simulink model "bf_ranger_indi"  (R2021a)
settings: Solver=VariableStepAuto  StartTime=0.0  StopTime=5  RelTol=1e-3
values from neighbouring files (symbols this model uses):
  am = 0.025    [ranger_sim.m]
  as = 0.08    [ranger_sim.m]
  G = [-10.67  10.67  0     0     0     0 0 ... (first row only)    [ranger_sim.m]
  G_inv = pinv(G)    [ranger_sim.m]
  G_thrust = [0 0 0 0 0 0 0 ... (first row only)    [ranger_sim.m]
  H_discr_den = cell2mat(Hd.den)    [ranger_sim.m]
  H_discr_num = cell2mat(Hd.num)    [ranger_sim.m]
  Kd = [10; 18; 18]    [ranger_sim.m]
  Kp = [4.1089; 4.7304; 7.36]    [ranger_sim.m]
  sample_time = 1/500    (= 0.002)    [ranger_sim.m]
undefined symbols (not defined in the file or in its folder): DiscIntNeverNeededParam
settings Model: Creator=AutomZ2-RG02B04  LastModifiedBy=AutomZ2-RG02A02
settings SolverCC: AlgebraicLoopSolver=TrustRegion

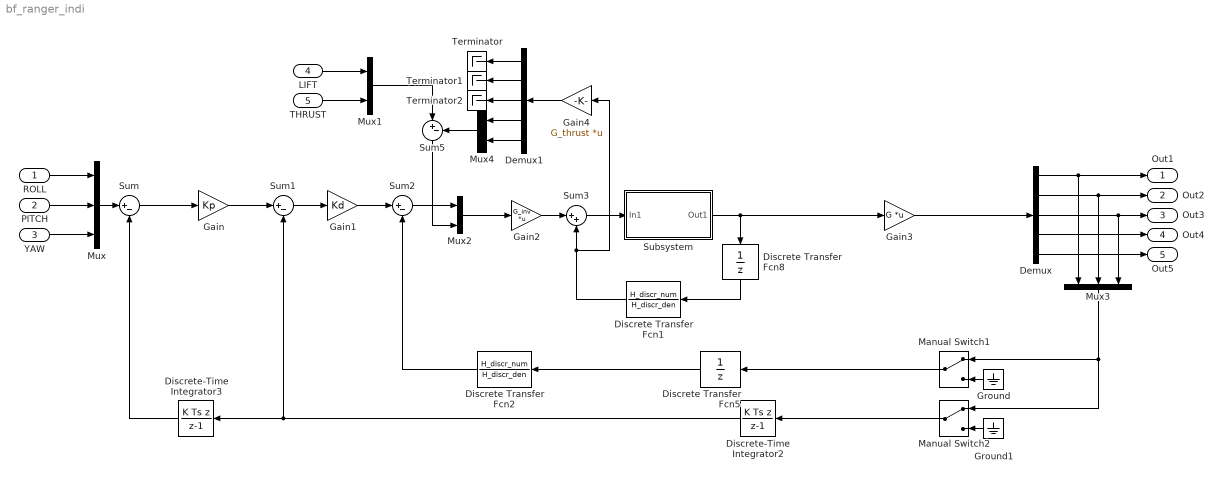
== system bf_ranger_indi ==
  ROLL : Inport
  PITCH : Inport  Port=2
  YAW : Inport  Port=3
  LIFT : Inport  Port=4
  THRUST : Inport  Port=5
  Demux : Demux  Outputs=5
  Demux1 : Demux  Outputs=5
  Discrete Transfer Fcn1 : DiscreteTransferFcn  Numerator=H_discr_num  Denominator=H_discr_den  SampleTime=sample_time
  Discrete Transfer Fcn2 : DiscreteTransferFcn  Numerator=H_discr_num  Denominator=H_discr_den  SampleTime=sample_time
  Discrete Transfer Fcn5 : DiscreteTransferFcn  Denominator=[1 0]  SampleTime=sample_time
  Discrete Transfer Fcn8 : DiscreteTransferFcn  Denominator=[1 0]  SampleTime=sample_time
  Discrete-Time Integrator2 : DiscreteIntegrator  IntegratorMethod=Integration: Backward Euler  SampleTime=sample_time  ICPrevOutput=DiscIntNeverNeededParam  ICPrevScaledInput=DiscIntNeverNeededParam
  Discrete-Time Integrator3 : DiscreteIntegrator  IntegratorMethod=Integration: Backward Euler  SampleTime=sample_time  ICPrevOutput=DiscIntNeverNeededParam  ICPrevScaledInput=DiscIntNeverNeededParam
  Gain : Gain  Gain=Kp
  Gain1 : Gain  Gain=Kd
  Gain2 : Gain  Gain=G_inv  Multiplication=Matrix(K*u)
  Gain3 : Gain  Gain=G  Multiplication=Matrix(K*u)
  Gain4 : Gain  Gain=G_thrust  Multiplication=Matrix(K*u)
  Ground : Ground
  Ground1 : Ground
  Manual Switch1 : ManualSwitch
  Manual Switch2 : ManualSwitch
  Mux : Mux  Inputs=3
  Mux1 : Mux  Inputs=2
  Mux2 : Mux  Inputs=2
  Mux3 : Mux  Inputs=3
  Mux4 : Mux  Inputs=2
  Subsystem : Subsystem
  Sum{,1..2,5} (4 alike) : Sum  Inputs=|+-
  Sum3 : Sum  Inputs=|++
  Terminator : Terminator
  Terminator1 : Terminator
  Terminator2 : Terminator
  Out1 : Outport
  Out2 : Outport  Port=2
  Out3 : Outport  Port=3
  Out4 : Outport  Port=4
  Out5 : Outport  Port=5
  wires:
  Sum/1 -> Gain/1
  Gain/1 -> Sum1/1
  Sum1/1 -> Gain1/1
  Gain1/1 -> Sum2/1
  Sum2/1 -> Mux2/1
  Gain2/1 -> Sum3/1
  Discrete Transfer Fcn5/1 -> Discrete Transfer Fcn2/1
  Discrete Transfer Fcn8/1 -> Discrete Transfer Fcn1/1
  Mux2/1 -> Gain2/1
  Sum3/1 -> Subsystem/1(In1)
  PITCH/1 -> Mux/2
  YAW/1 -> Mux/3
  Mux/1 -> Sum/1
  LIFT/1 -> Mux1/1
  THRUST/1 -> Mux1/2
  Demux/1 -> Mux3/1, Out1/1
  Demux/2 -> Mux3/2, Out2/1
  Demux/3 -> Out3/1, Mux3/3
  Demux/4 -> Out4/1
  Demux/5 -> Out5/1
  ROLL/1 -> Mux/1
  Subsystem/1(Out1) -> Discrete Transfer Fcn8/1, Gain3/1
  Gain3/1 -> Demux/1
  Discrete Transfer Fcn2/1 -> Sum2/2
  Discrete-Time Integrator2/1 -> Discrete-Time Integrator3/1, Sum1/2
  Discrete-Time Integrator3/1 -> Sum/2
  Discrete Transfer Fcn1/1 -> Gain4/1, Sum3/2
  Mux1/1 -> Sum5/1
  Sum5/1 -> Mux2/2
  Manual Switch1/1 -> Discrete Transfer Fcn5/1
  Manual Switch2/1 -> Discrete-Time Integrator2/1
  Mux3/1 -> Manual Switch2/1, Manual Switch1/1
  Ground/1 -> Manual Switch1/2
  Ground1/1 -> Manual Switch2/2
  Demux1/3 -> Terminator2/1
  Demux1/4 -> Mux4/1
  Demux1/2 -> Terminator1/1
  Gain4/1 -> Demux1/1
  Mux4/1 -> Sum5/2
  Demux1/5 -> Mux4/2
  Demux1/1 -> Terminator/1

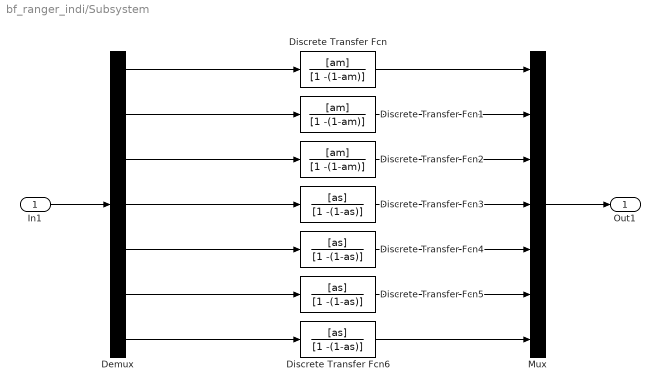
== system bf_ranger_indi/Subsystem ==
  In1 : Inport
  Demux : Demux  Outputs=7
  Discrete Transfer Fcn : DiscreteTransferFcn  Numerator=[am]  Denominator=[1 -(1-am)]  SampleTime=sample_time
  Discrete Transfer Fcn1 : DiscreteTransferFcn  Numerator=[am]  Denominator=[1 -(1-am)]
  Discrete Transfer Fcn2 : DiscreteTransferFcn  Numerator=[am]  Denominator=[1 -(1-am)]
  Discrete Transfer Fcn{3..6} (4 alike) : DiscreteTransferFcn  Numerator=[as]  Denominator=[1 -(1-as)]
  Mux : Mux  Inputs=7
  Out1 : Outport
  wires:
  Discrete Transfer Fcn/1 -> Mux/1
  Discrete Transfer Fcn1/1 -> Mux/2
  Demux/2 -> Discrete Transfer Fcn1/1
  Discrete Transfer Fcn2/1 -> Mux/3
  Demux/3 -> Discrete Transfer Fcn2/1
  Demux/5 -> Discrete Transfer Fcn4/1
  Discrete Transfer Fcn3/1 -> Mux/4
  Demux/4 -> Discrete Transfer Fcn3/1
  Discrete Transfer Fcn4/1 -> Mux/5
  Discrete Transfer Fcn5/1 -> Mux/6
  Demux/6 -> Discrete Transfer Fcn5/1
  Discrete Transfer Fcn6/1 -> Mux/7
  Demux/7 -> Discrete Transfer Fcn6/1
  In1/1 -> Demux/1
  Demux/1 -> Discrete Transfer Fcn/1
  Mux/1 -> Out1/1
